simulink model "sim_file2"  (Simulink 9.2)
settings: Solver=VariableStepAuto  StartTime=0.0  StopTime=10.0  RelTol=1e-3
values from neighbouring files (symbols this model uses):
  C_ctl = [0 0 114594.2 0.001 -114594.2 -0.001]    [cntl_sys.mat]    (also in main_cntl.m = [0 , 0  , Ks , ds , -Ks , -ds  ])
  ctl = lqr(sys_ctl,Q,R)    [main_cntl.m]
  sys_ctl = ss(A,B,C1,0)    [main_cntl.m]    (also in main_tf_8.m = ss(A,B,C,0))
settings Model: Creator=eshojaei  LastModifiedBy=eshojaei
settings DataIOCC: LimitDataPoints=off  SaveFormat=Dataset  SignalLoggingSaveFormat=Dataset
settings OptimizationCC: LifeSpan=auto
settings DebuggingCC: UnderspecifiedInitializationDetection=Simplified  MergeDetectMultiDrivingBlocksExec=error  FcnCallInpInsideContextMsg=error  StateNameClashWarn=none  SFUnexpectedBacktrackingDiag=error  SFNoUnconditionalDefaultTransitionDiag=error  SFExecutionAtInitializationDiag=warning
settings HardwareCC: ProdBitPerPointer=64  ProdBitPerSizeT=64  ProdBitPerPtrDiffT=64  ProdLargestAtomicFloat=Float  ProdIntDivRoundTo=Zero  ProdEndianess=LittleEndian  ProdWordSize=64  ProdHWDeviceType=Intel->x86-64 (Windows64)
settings ModelReferenceCC: PropagateSignalLabelsOutOfModel=on
settings SFSimCC: SimUseLocalCustomCode=on
settings RTWCC: RTWUseLocalCustomCode=on
settings CodeAppCC: StateflowObjectComments=off
settings GRTTargetCC: TargetLangStandard=C99 (ISO)  GeneratePreprocessorConditionals=Use local settings  CombineOutputUpdateFcns=on  GRTInterface=off
settings ConfigComp: CovMetricSettings=dwe  CovHtmlReporting=off  CovSaveCumulativeToWorkspaceVar=off  CovSaveSingleToWorkspaceVar=off  CovExternalEMLEnable=on

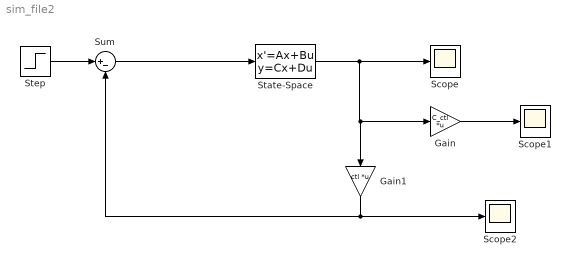
== system sim_file2 ==
  Gain : Gain  Gain=C_ctl  Multiplication=Matrix(K*u)
  Gain1 : Gain  Gain=ctl  Multiplication=Matrix(K*u)
  Scope : Scope
  Scope1 : Scope
  Scope2 : Scope
  State-Space : StateSpace  A=sys_ctl.A  B=sys_ctl.B  C=sys_ctl.C  D=sys_ctl.D  InitialCondition=0
  Step : Step  Time=.1  After=10  SampleTime=0
  Sum : Sum  Inputs=|+-
  wires:
  Gain/1 -> Scope1/1
  Sum/1 -> State-Space/1
  Step/1 -> Sum/1
  State-Space/1 -> Scope/1, Gain/1, Gain1/1
  Gain1/1 -> Sum/2, Scope2/1
